simulink model "Q2_3"  (R2020b)
settings: Solver=VariableStepAuto  StartTime=0.0  StopTime=100.0  RelTol=1e-3
settings Model: Creator=kushagrakhatwani  LastModifiedBy=kushagrakhatwani

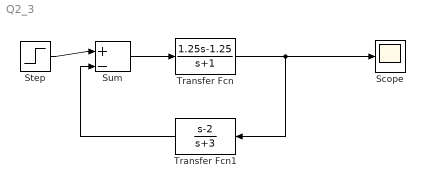
== system Q2_3 ==
  Scope : Scope
  Step : Step  Time=0  SampleTime=0
  Sum : Sum  Inputs=|+-
  Transfer Fcn : TransferFcn  Numerator=[1.25 -1.25]  Denominator=[1 1]
  Transfer Fcn1 : TransferFcn  Numerator=[1 -2]  Denominator=[1 3]
  wires:
  Step/1 -> Sum/1
  Sum/1 -> Transfer Fcn/1
  Transfer Fcn1/1 -> Sum/2
  Transfer Fcn/1 -> Transfer Fcn1/1, Scope/1
